simulink model "EnvP_VD"  (R2016b)
settings: configuration reference "CodeGenConfigSet" (kept outside this file)
values from neighbouring files (symbols this model uses):
  EnvP_facPT1_C = Calibration.Parameter    [init_EnvP_VD.m]
  EnvP_pTransStgDfl_C = Calibration.Parameter    [init_EnvP_VD.m]
  EnvP_RmpSlpNeg_C = Calibration.Parameter    [init_EnvP_VD.m]
  EnvP_RmpSlpPos_C = Calibration.Parameter    [init_EnvP_VD.m]
  SigTst_pEnvP_C = Calibration.Parameter    [init_EnvP_VD.m]
  SigTst_swtEnvP_C = Calibration.Parameter    [init_EnvP_VD.m]
undefined symbols (not defined in the file or in its folder): CEngDst_switch_conv, EnvP_VD_DT, Switch_conv
libraries: CXLib x4
settings Model: Creator=lenovo  LastModifiedBy=lenovo
settings ConfigSetRef: SourceLocation=Base Workspace

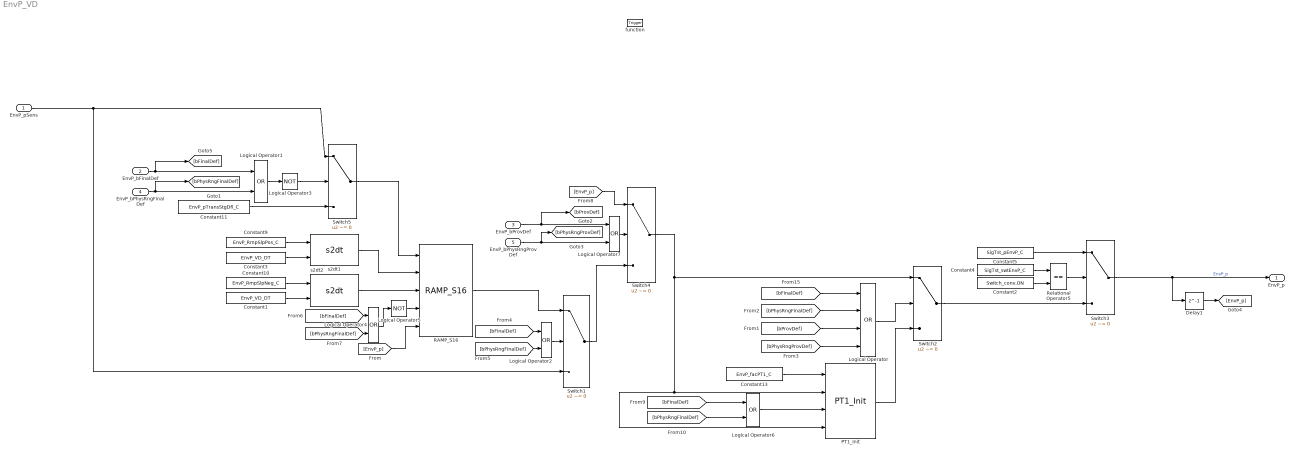
== system EnvP_VD ==
  EnvP_pSens : Inport  Tag=kPa  Description=Raw physical value  OutMin=0  OutMax=1200  OutDataTypeStr=AirPressure_kPa
  EnvP_bFinalDef : Inport  Description=Environment pressure sensor finally defect flag  Port=2  OutMin=0  OutMax=1  OutDataTypeStr=boolean
  EnvP_bProvDef : Inport  Description=Environment pressure sensor temporary defect flag  Port=3  OutMin=0  OutMax=1  OutDataTypeStr=boolean
  EnvP_bPhysRngFinalDef : Inport  Description=Environment pressure sensor physical range finally defect  Port=4  OutMin=0  OutMax=1  OutDataTypeStr=boolean
  EnvP_bPhysRngProvDef : Inport  Description=Environment pressure sensor physical range temporary defect  Port=5  OutMin=0  OutMax=1  OutDataTypeStr=boolean
  function : TriggerPort  TriggerType=function-call  VariantControl=Variant
  Constant1 : Constant  Value=EnvP_VD_DT  OutDataTypeStr=Inherit: Inherit via back propagation
  Constant10 : Constant  RequirementInfo={'other' 'CEngDsT_requirements.doc' '@Simulink_requirement_item_8' 'true' '冷却水温故障时斜坡至默认值' '' } %GIDa_8b51e30d_3fed_4578_b862_07a9192f7094  Value=EnvP_RmpSlpNeg_C  SampleTime=-1
  Constant11 : Constant  RequirementInfo={'other' 'CEngDsT_requirements.doc' '@Simulink_requirement_item_8' 'true' '冷却水温故障时斜坡至默认值' '' } %GIDa_e17b814d_2c78_4849_a646_c2bfce48f8cb  Value=EnvP_pTransStgDfl_C  SampleTime=-1
  Constant13 : Constant  Value=EnvP_facPT1_C  SampleTime=-1
  Constant2 : Constant  RequirementInfo={'other' 'APP_requirements.doc' '@Simulink_requirement_item_25' 'true' '手动开关' '' } %GIDa_97a72ce1_7d44_4d59_a9db_9e24c49048f3  Value=Switch_conv.ON  OutDataTypeStr=Inherit: Inherit via back propagation
  Constant3 : Constant  Value=EnvP_VD_DT  OutDataTypeStr=Inherit: Inherit via back propagation
  Constant4 : Constant  RequirementInfo={'other' 'CEngDsT_requirements.doc' '@Simulink_requirement_item_6' 'true' '手动冷却水温值' '' } %GIDa_78b71db0_407f_463c_b40a_58853ac02589  Value=SigTst_swtEnvP_C  SampleTime=-1
  Constant5 : Constant  RequirementInfo={'other' 'CEngDsT_requirements.doc' '@Simulink_requirement_item_6' 'true' '手动冷却水温值' '' } %GIDa_d59b62ca_b964_47d3_9302_fbd97b0d16b6  Value=SigTst_pEnvP_C  SampleTime=-1
  Constant9 : Constant  RequirementInfo={'other' 'CEngDsT_requirements.doc' '@Simulink_requirement_item_8' 'true' '冷却水温故障时斜坡至默认值' '' } %GIDa_24e3dd61_05cb_4b09_9b03_8807a1549053  Value=EnvP_RmpSlpPos_C  SampleTime=-1
  Delay1 : Delay  DialogController=Simulink.DDGSource  DelayLength=1  InitialCondition=0
  Logical Operator : Logic  Operator=OR  Inputs=4  OutDataTypeStr=boolean
  Logical Operator{1..2,4,6..7} (5 alike) : Logic  Operator=OR  OutDataTypeStr=boolean
  Logical Operator3 : Logic  Operator=NOT  AllPortsSameDT=off  OutDataTypeStr=boolean
  Logical Operator5 : Logic  Operator=NOT  AllPortsSameDT=off  OutDataTypeStr=boolean
  PT1_Init : CXLib/PT1_Init
  RAMP_S16 : CXLib/RAMP_S16  RequirementInfo={'other' 'CEngDsT_requirements.doc' '@Simulink_requirement_item_8' 'true' '冷却水温故障时斜坡至默认值' '' } %GIDa_d5bc8cc9_487c_4666_8fca_402446b727fb
  Relational Operator5 : RelationalOperator  Operator===  OutDataTypeStr=boolean  RndMeth=Simplest  InputSameDT=on
  Switch1 : Switch  Criteria=u2 ~= 0  InputSameDT=on
  Switch2 : Switch  RequirementInfo={'other' 'CEngDsT_requirements.doc' '@Simulink_requirement_item_5' 'true' '冷却水温滤波去抖动' '' } %GIDa_890eeffe_50f1_4e6b_bd17_7d653fc513c6  Criteria=u2 ~= 0  InputSameDT=on
  Switch3 : Switch  RequirementInfo={'other' 'CEngDsT_requirements.doc' '@Simulink_requirement_item_6' 'true' '手动冷却水温值' '' } %GIDa_9621f7e7_909d_4b84_994e_39f744445bbc  Criteria=u2 ~= 0  Threshold=CEngDst_switch_conv.OFF  InputSameDT=on
  Switch4 : Switch  Criteria=u2 ~= 0  InputSameDT=on
  Switch5 : Switch  Criteria=u2 ~= 0  InputSameDT=on
  s2dt1 : CXLib/s2dt
  s2dt2 : CXLib/s2dt
  EnvP_p : Outport  Tag=kPa  Description=Barometric pressure  OutMin=0  OutMax=3276  OutDataTypeStr=AirPressure_kPa
  wires:
  [EnvP_p] -> Switch4/1
  s2dt2/1 -> RAMP_S16/3
  Constant1/1 -> s2dt2/2
  Constant3/1 -> s2dt1/2
  s2dt1/1 -> RAMP_S16/2
  [EnvP_p] -> RAMP_S16/5
  Delay1/1 -> [EnvP_p]
  Logical Operator6/1 -> PT1_Init/3
  [bPhysRngFinalDef] -> Logical Operator6/2
  [bFinalDef] -> Logical Operator6/1
  Logical Operator5/1 -> RAMP_S16/4
  [bPhysRngFinalDef] -> Logical Operator4/2
  [bFinalDef] -> Logical Operator4/1
  [bPhysRngFinalDef] -> Logical Operator2/2
  [bFinalDef] -> Logical Operator2/1
  Constant2/1 -> Relational Operator5/2
  Constant4/1 -> Relational Operator5/1
  Relational Operator5/1 -> Switch3/2
  [bPhysRngProvDef] -> Logical Operator/4
  [bProvDef] -> Logical Operator/3
  [bPhysRngFinalDef] -> Logical Operator/2
  [bFinalDef] -> Logical Operator/1
  EnvP_bPhysRngProvDef/1 -> Logical Operator7/2, [bPhysRngProvDef]
  EnvP_bProvDef/1 -> Logical Operator7/1, [bProvDef]
  EnvP_bFinalDef/1 -> Logical Operator1/1, [bFinalDef]
  EnvP_bPhysRngFinalDef/1 -> Logical Operator1/2, [bPhysRngFinalDef]
  PT1_Init/1 -> Switch2/3
  RAMP_S16/1 -> Switch1/1
  Switch5/1 -> RAMP_S16/1
  Constant13/1 -> PT1_Init/1
  Constant10/1 -> s2dt2/1
  Constant9/1 -> s2dt1/1
  Constant5/1 -> Switch3/1
  Logical Operator4/1 -> Logical Operator5/1
  Logical Operator2/1 -> Switch1/2
  Logical Operator7/1 -> Switch4/2
  Logical Operator3/1 -> Switch5/2
  Logical Operator1/1 -> Logical Operator3/1
  Constant11/1 -> Switch5/3
  Switch3/1 -> EnvP_p/1, Delay1/1  "EnvP_p"
  Switch2/1 -> Switch3/3
  Logical Operator/1 -> Switch2/2
  Switch1/1 -> Switch4/3
  Switch4/1 -> Switch2/1, PT1_Init/4, PT1_Init/2
  EnvP_pSens/1 -> Switch5/1, Switch1/3
